simulink model "temp_fusion"  (R2018a)
settings: Solver=VariableStepAuto  StartTime=0.0  StopTime=10  RelTol=1e-3
libraries: simulink x1, sharedTrackingLibrary x1
settings Model: Creator=cnxsoftware  LastModifiedBy=Zzimon

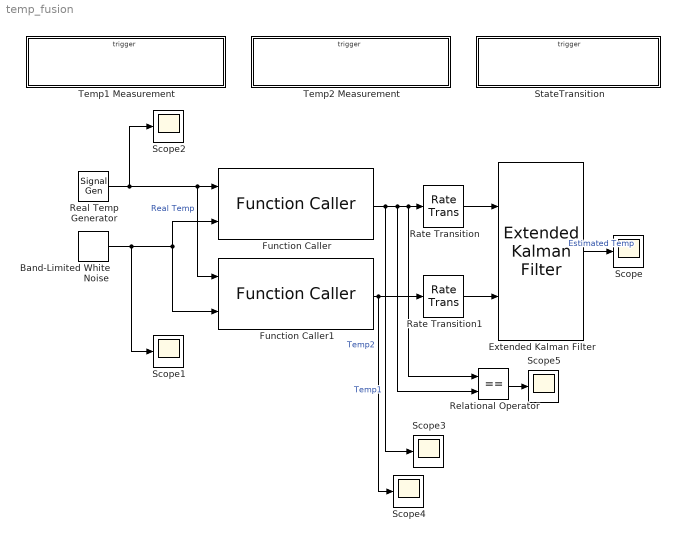
== system temp_fusion ==
  Band-Limited White Noise : simulink/Sources/Band-Limited White Noise  Cov=[0.00001]  Ts=0.001  seed=[23341]
  Extended Kalman Filter : sharedTrackingLibrary/Extended Kalman Filter  StateTransitionFcn=stateTransitionFcn  HasStateTransitionJacobianFcn=off  HasAdditiveProcessNoise=Nonadditive  ProcessNoise=0.5  HasTimeVaryingProcessNoise=off  HasStateTransitionFcnExtraArgument=0  InitialState=0  InitialStateCovariance=1  MeasurementFcn1=Temp1MeasurementFcn  HasMeasurementJacobianFcn1=off  HasMeasurementEnablePort1=off  HasAdditiveMeasurementNoise1=Nonadditive  MeasurementNoise1=0.2  HasTimeVaryingMeasurementNoise1=off  HasMeasurementFcnExtraArgument1=0  MeasurementFcn2=Temp2MeasurementFcn  HasMeasurementJacobianFcn2=off  HasMeasurementEnablePort2=off  HasAdditiveMeasurementNoise2=Nonadditive  MeasurementNoise2=0.2  HasTimeVaryingMeasurementNoise2=off  HasMeasurementFcnExtraArgument2=0  MeasurementFcn3=myMeasurementFcn  HasMeasurementJacobianFcn3=off  HasMeasurementEnablePort3=off  HasAdditiveMeasurementNoise3=Additive  MeasurementNoise3=1  HasTimeVaryingMeasurementNoise3=off  HasMeasurementFcnExtraArgument3=0  MeasurementFcn4=myMeasurementFcn  HasMeasurementJacobianFcn4=off  HasMeasurementEnablePort4=off  HasAdditiveMeasurementNoise4=Additive  MeasurementNoise4=1  HasTimeVaryingMeasurementNoise4=off  HasMeasurementFcnExtraArgument4=0  MeasurementFcn5=myMeasurementFcn  HasMeasurementJacobianFcn5=off  HasMeasurementEnablePort5=off  HasAdditiveMeasurementNoise5=Additive  MeasurementNoise5=1  HasTimeVaryingMeasurementNoise5=off  HasMeasurementFcnExtraArgument5=0  EnableMultirate=off  StateTransitionFcnSampleTime=1  MeasurementFcn1SampleTime=1  MeasurementFcn2SampleTime=1  MeasurementFcn3SampleTime=1  MeasurementFcn4SampleTime=1  MeasurementFcn5SampleTime=1  UseCurrentEstimator=on  OutputStateCovariance=off  DataType=double  SampleTime=0.01  NumberOfMeasurements=2
      settings: SourceProductName=Control System Toolbox  SourceProductBaseCode=CT
  Function Caller : FunctionCaller  FunctionPrototype=y = Temp1MeasurementFcn(x,v)
  Function Caller1 : FunctionCaller  FunctionPrototype=y = Temp2MeasurementFcn(x,v)
  Rate Transition : RateTransition
  Rate Transition1 : RateTransition
  Real Temp Generator : SignalGenerator  Units=rad/sec
  Relational Operator : RelationalOperator  Operator===  OutDataTypeStr=boolean  RndMeth=Simplest
  Scope{,1..5} (6 alike) : Scope
  StateTransition : Subsystem  TreatAsAtomicUnit=on
  Temp1 Measurement : Subsystem  TreatAsAtomicUnit=on
  Temp2 Measurement : Subsystem  TreatAsAtomicUnit=on
  wires:
  Real Temp Generator/1 -> Scope2/1, Function Caller1/1, Function Caller/1  "Real Temp"
  Band-Limited White Noise/1 -> Scope1/1, Function Caller/2, Function Caller1/2
  Function Caller/1 -> Scope3/1, Relational Operator/2, Relational Operator/1, Rate Transition/1  "Temp1"
  Function Caller1/1 -> Scope4/1, Rate Transition1/1  "Temp2"
  Extended Kalman Filter/1 -> Scope/1  "Estimated Temp"
  Rate Transition/1 -> Extended Kalman Filter/1
  Rate Transition1/1 -> Extended Kalman Filter/2
  Relational Operator/1 -> Scope5/1

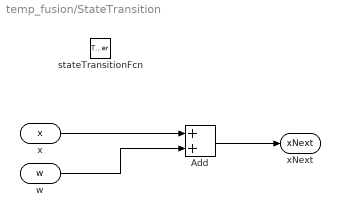
== system temp_fusion/StateTransition ==
  stateTransitionFcn : TriggerPort  TriggerType=function-call  IsSimulinkFunction=on  FunctionName=stateTransitionFcn  FunctionVisibility=scoped  VariantControl=(inherit)
  Add : Sum
  x : ArgIn  DisableCoverage=on  ArgumentName=x
  w : ArgIn  Port=2  ArgumentName=w
  xNext : ArgOut  DisableCoverage=on  ArgumentName=xNext
  wires:
  w/1 -> Add/2
  Add/1 -> xNext/1
  x/1 -> Add/1

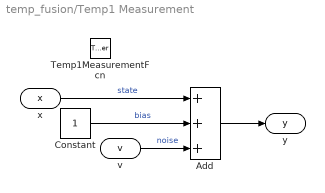
== system temp_fusion/Temp1 Measurement ==
  Temp1MeasurementFcn : TriggerPort  TriggerType=function-call  IsSimulinkFunction=on  FunctionName=Temp1MeasurementFcn  FunctionVisibility=scoped  VariantControl=(inherit)
  Add : Sum  Inputs=+++
  Constant : Constant
  x : ArgIn  DisableCoverage=on  ArgumentName=x
  v : ArgIn  Port=2  ArgumentName=v
  y : ArgOut  DisableCoverage=on  ArgumentName=y
  wires:
  Add/1 -> y/1
  x/1 -> Add/1  "state"
  Constant/1 -> Add/2  "bias"
  v/1 -> Add/3  "noise"

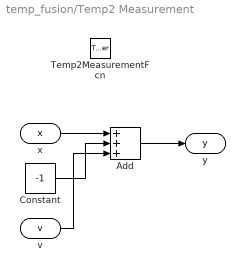
== system temp_fusion/Temp2 Measurement ==
  Temp2MeasurementFcn : TriggerPort  TriggerType=function-call  IsSimulinkFunction=on  FunctionName=Temp2MeasurementFcn  FunctionVisibility=scoped  VariantControl=(inherit)
  Add : Sum  Inputs=+++
  Constant : Constant  Value=-1
  x : ArgIn  DisableCoverage=on  ArgumentName=x
  v : ArgIn  Port=2  ArgumentName=v
  y : ArgOut  DisableCoverage=on  ArgumentName=y
  wires:
  v/1 -> Add/3
  Add/1 -> y/1
  Constant/1 -> Add/2
  x/1 -> Add/1
